simulink model "vehicle_model"  (R2021b)
settings: Solver=ode23tb  StartTime=0  StopTime=181.45  FixedStep=1e-5  RelTol=2e-1
InitFcn:
  | param_v1_script;
  | Ts=0.01;
  | scenario_generator;
  | Regen_on=0;
  | v_nom=10;
  | load('eq_udds.mat')
  | %load('eq_nedc.mat')
values from neighbouring files (symbols this model uses):
  b = 1.504    [dynamics_wheel.m]    (also in param_v1_script.m = Simulink.Parameter)
  BattChargeMax = 4.8    [param_v1_script.m]
  Battery = struct    [param_v1_script.m]
  BattSocInit = 0.75    [param_v1_script.m]
  BattTempInit = 25    [param_v1_script.m]
  BrkPrsMax = 5.0E+6    (= 5000000)    [param_v1_script.m]
  car = vehicle(scenario,'ClassID',1,'Position',[x_ego y_ego 0], 'Yaw' ,0,     'Length',3,'Width',2,'Height',1.6)    [scenario_generator.m]
  curvature = (DX.*D2Y - DY.*D2X) ./(DX.^2+DY.^2).^(3/2)    [ref_generator.m]
  direction = ones(length(gradbp),1)    [ref_generator.m]
  disk_abore = 0.05    [param_v1_script.m]
  Eb_init = 54.28*1000*3600    (= 195408000)    [param_v1_script.m]
  efficiency_table = [86.7 86.7 86.7 86.7 86.7 86.7 86.7 86.7 86.7 86.7 86.7 86.7 86.7 86.7     86.7 ... (first row only)    [param_v1_script.m]
  eta_i = 1    [param_v1_script.m]
  gradbp = distbp    [ref_generator.m]
  Jmotor = Simulink.Parameter    [param_v1_script.m]
  k = Simulink.Parameter    [param_v1_script.m]
  L = 30000    [scenario_generator.m]
  losses_table = [0 0 0 0 0 0 0 0 0 0 0 0 0 0 0 ... (first row only)    [param_v1_script.m]
  m = 3152    [param_v1_script.m]
  MaxChrgCurrLim = Simulink.Parameter    [param_v1_script.m]
  MaxDchrgCurrLim = Simulink.Parameter    [param_v1_script.m]
  MinCellVoltDchrgCurrentLim_BP = [2.5; 2.75; 3]    [param_v1_script.m]
  MinCellVoltDchrgCurrentLim_Table = [0 0.5 1]    [param_v1_script.m]
  MotSpd = [0 1600 3200 4477.56 4800 6400 8000 9600 11200 12800 14400 16000            ]    [param_v1_script.m]
  MotTrq = [450 450 450 450 419.771162404874 314.828371803655 251.862697442924            209.885581202437 179.901926744946 157.414185901828 139.923720801625            125.931348721462]    [param_v1_script.m]
  mu_kinetic = 0.2    [param_v1_script.m]
  Nd = 12    [param_v1_script.m]
  Ndiff = Simulink.Parameter    [param_v1_script.m]
  Np_Module = 31    [param_v1_script.m]
  Ns_Module = 24    [param_v1_script.m]
  num_pads = 2    [param_v1_script.m]
  NumModules = 4    [param_v1_script.m]
  psi_o = thetaRefs(1)*(pi/180)    [ref_generator.m]
  RegenBrkCutOff = [0 1]    [param_v1_script.m]
  RegenBrkSpd_bpt = [5 9]    [param_v1_script.m]
  Rm = 0.177    [param_v1_script.m]
  rw = 0.419    [param_v1_script.m]
  scenario = drivingScenario('SampleTime',0.1','StopTime',60)    [scenario_generator.m]
  SOCInit = 0.75    [param_v1_script.m]
  SOE_init = SOCInit    (= 0.75)    [param_v1_script.m]
  T_eff_bp = [0 32.142857142857146 64.285714285714292 96.428571428571431              128.57142857142858 160.71428571428572 192.85714285714286 225              257.14285714285717 289.28571428571428 321.42857142857144 353.57142857142856              385.71428571428572 417.85714285714283 450]    [param_v1_script.m]
  thetaRefs = smooth(gradbp,thetaRef)    [ref_generator.m]
  threshld = 50    [scenario_generator.m]
  VEH = struct    [dynamics_wheel.m]
  w_eff_bp = [0 1600 3200 4477.56 4800 6400 8000 9600 11200 12800 14400 16000              ]    [param_v1_script.m]
  xRef2s = smooth(gradbp,xRef2)    [ref_generator.m]
  yRef2s = smooth(gradbp,yRef2)    [ref_generator.m]
undefined symbols (not defined in the file or in its folder): DiscIntNeverNeededParam, InertFrm
libraries: simulink x11, autolibsharedcoupling x10, autolibshared x5, autolibutils x4, autolibshareddiff x3, sharedtransform x3, vehdynlibdriver x3, simulink_extras x3, sharedTrackingLibrary x2, vehdynlibtirecommon x2, vehdynlibtire x2, vehdynlibdrivercommon x2
(part 6 of 6)

== system vehicle_model/Passenger Car/Subsystem1/Subsystem1/Longitudinal Wheels 4DOF/Axle Forces/Bicycle/Wheel to Body Transform ==
  Forces : Inport  PortDimensions=[3,1]  Partition=on  PartitionDimension=2  PartitionWidth=1  PartitionOffset=0
  WheelAngles : Inport  Port=2  Partition=on  PartitionDimension=2  PartitionWidth=1  PartitionOffset=0
  Demux1 : Demux  Outputs=3
  Divide1 : Product  Inputs=**  Multiplication=Matrix(*)
  For Each : ForEach  DisableCoverage=on
  Rotation Angles to Direction Cosine Matrix : sharedtransform/Rotation Angles to Direction Cosine Matrix  rotationOrder=ZYX  aMode=2
      settings: SourceProductBaseCode=AE,PW,DR,MT,UV,VE
  Selector : Selector  InputPortWidth=3  IndexOptions=Index vector (dialog)  Indices=[3 2 1]  OutputSizes=1
  Fx : Outport  ConcatenationDimension=1  VectorParamsAs1DForOutWhenUnconnected=off
  Fy : Outport  Port=2  ConcatenationDimension=1  VectorParamsAs1DForOutWhenUnconnected=off
  Fz : Outport  Port=3  ConcatenationDimension=1  VectorParamsAs1DForOutWhenUnconnected=off
  wires:
  Selector/1 -> Rotation Angles to Direction Cosine Matrix/1
  WheelAngles/1 -> Selector/1
  Forces/1 -> Divide1/2
  Rotation Angles to Direction Cosine Matrix/1 -> Divide1/1
  Demux1/3 -> Fz/1
  Demux1/2 -> Fy/1
  Demux1/1 -> Fx/1
  Divide1/1 -> Demux1/1

== system vehicle_model/Passenger Car/Subsystem1/Subsystem1/Longitudinal Wheels 4DOF/Axle Forces/Dual/Wheel Angles ==
  Front : Inport
  Camber : Inport  Port=2
  Add1 : Sum
  Add2 : Sum
  Constant1 : Constant  Value=pi
  Constant2 : Constant  Value=[pi;0;pi;0].*0+[0;pi;0;pi].*.0
  Constant3 : Constant  Value=ones(1,4).*0
  Reshape : Reshape  OutputDimensionality=Row vector (2-D)
  Reshape1 : Reshape  OutputDimensionality=Row vector (2-D)
  Reshape2 : Reshape  OutputDimensionality=Row vector (2-D)
  Vector Concatenate3 : Concatenate  NumInputs=3  Mode=Multidimensional array
  Vehicle : Outport  VectorParamsAs1DForOutWhenUnconnected=off
  wires:
  Constant1/1 -> Add2/2
  Reshape/1 -> Vector Concatenate3/3
  Reshape2/1 -> Vector Concatenate3/2
  Front/1 -> Add1/1
  Add2/1 -> Reshape1/1
  Add1/1 -> Reshape/1
  Constant3/1 -> Reshape2/1
  Reshape1/1 -> Vector Concatenate3/1
  Constant2/1 -> Add1/2
  Camber/1 -> Add2/1
  Vector Concatenate3/1 -> Vehicle/1

== system vehicle_model/Passenger Car/Subsystem1/Subsystem1/Longitudinal Wheels 4DOF/Axle Forces/Dual/Wheel to Body Transform ==
  Forces : Inport  PortDimensions=[3,1]  Partition=on  PartitionDimension=2  PartitionWidth=1  PartitionOffset=0
  WheelAngles : Inport  Port=2  Partition=on  PartitionDimension=2  PartitionWidth=1  PartitionOffset=0
  Demux1 : Demux  Outputs=3
  Divide1 : Product  Inputs=**  Multiplication=Matrix(*)
  For Each : ForEach  DisableCoverage=on
  Rotation Angles to Direction Cosine Matrix : sharedtransform/Rotation Angles to Direction Cosine Matrix  rotationOrder=ZYX  aMode=2
      settings: SourceProductBaseCode=AE,PW,DR,MT,UV,VE
  Selector : Selector  InputPortWidth=3  IndexOptions=Index vector (dialog)  Indices=[3 2 1]  OutputSizes=1
  Fx : Outport  ConcatenationDimension=1  VectorParamsAs1DForOutWhenUnconnected=off
  Fy : Outport  Port=2  ConcatenationDimension=1  VectorParamsAs1DForOutWhenUnconnected=off
  Fz : Outport  Port=3  ConcatenationDimension=1  VectorParamsAs1DForOutWhenUnconnected=off
  wires:
  Divide1/1 -> Demux1/1
  Demux1/1 -> Fx/1
  Demux1/2 -> Fy/1
  Demux1/3 -> Fz/1
  Rotation Angles to Direction Cosine Matrix/1 -> Divide1/1
  Forces/1 -> Divide1/2
  WheelAngles/1 -> Selector/1
  Selector/1 -> Rotation Angles to Direction Cosine Matrix/1

== system vehicle_model/Passenger Car/Subsystem1/Subsystem1/Longitudinal Wheels 4DOF/Tires/MF/scale factors with friction ==
  lamda_mu_x : Inport
  lamda_mu_y : Inport  Port=2
  0 : Constant  Value=[zeros(1,numWheels)]  VectorParams1D=off
  Reshape : Reshape  OutputDimensionality=Row vector (2-D)  OutputDimensions=[1,numWheels]
  Reshape1 : Reshape  OutputDimensionality=Row vector (2-D)  OutputDimensions=[1,numWheels]
  Signal Specification3 : SignalSpecification  Unit=1
  Vector Concatenate : Concatenate  NumInputs=5  Mode=Multidimensional array
  ones : Constant  Value=[ones(23,numWheels)]  VectorParams1D=off
  ones2 : Constant  Value=ones(1,numWheels)  VectorParams1D=off
  lambdas : Outport  Unit=1  VectorParamsAs1DForOutWhenUnconnected=off
  wires:
  lamda_mu_y/1 -> Reshape1/1
  lamda_mu_x/1 -> Reshape/1
  ones2/1 -> Vector Concatenate/1  "lambda_Fz0"
  Vector Concatenate/1 -> Signal Specification3/1
  ones/1 -> Vector Concatenate/5
  0/1 -> Vector Concatenate/4  "lamda_mu_V"
  Reshape1/1 -> Vector Concatenate/3
  Reshape/1 -> Vector Concatenate/2
  Signal Specification3/1 -> lambdas/1

== system vehicle_model/Passenger Car/Subsystem1/Subsystem1/Longitudinal Wheels 4DOF/Velocity and Vertical Load/Bicycle/Bicycle Fz ==
  Bus Element In1 : Inport  PortName=VehFdbk
  Add : Sum
  Bus Selector : BusSelector  OutputSignals=BdyFrm.Forces.Tires.FrntTire.Fz,BdyFrm.Forces.Tires.RearTire.Fz
  Cont LPF : autolibutils/Cont LPF  wc=100*2*pi*ones(4,1)  aMode=2
      settings: SourceProductBaseCode=PW,DR,MT,UV,VE
  Saturation : Saturate  UpperLimit=10e3*ones(4,1)  LowerLimit=100*ones(4,1)  ZeroCross=off
  Unsprung Mass : Constant  Value=[0 0 80 80].*9.81
  Vector Concatenate : Concatenate  NumInputs=4
  Out1 : Outport  PortDimensions=4  VectorParamsAs1DForOutWhenUnconnected=off
  wires:
  Vector Concatenate/1 -> Saturation/1
  Saturation/1 -> Cont LPF/1
  Cont LPF/1 -> Add/1
  Bus Element In1/1 -> Bus Selector/1
  Bus Selector/1 -> Vector Concatenate/2, Vector Concatenate/1  "<Fz>"
  Bus Selector/2 -> Vector Concatenate/3, Vector Concatenate/4  "<Fz>"
  Unsprung Mass/1 -> Add/2
  Add/1 -> Out1/1

== system vehicle_model/Passenger Car/Subsystem1/Subsystem1/Longitudinal Wheels 4DOF/Velocity and Vertical Load/Bicycle/Bicycle V ==
  In1 : Inport
  Bus Selector : BusSelector  OutputSignals=BdyFrm.FrntAxl.Vel.xdot,BdyFrm.FrntAxl.Vel.ydot,BdyFrm.FrntAxl.Vel.zdot
  Bus Selector3 : BusSelector  OutputSignals=BdyFrm.RearAxl.Vel.xdot,BdyFrm.RearAxl.Vel.ydot,BdyFrm.RearAxl.Vel.zdot
  Mux : Mux  Inputs=3
  Mux1 : Mux  Inputs=3
  Vector Concatenate1 : Concatenate  NumInputs=4  Mode=Multidimensional array  ConcatenateDimension=2
  Out1 : Outport  PortDimensions=[3,4]  VectorParamsAs1DForOutWhenUnconnected=off
  wires:
  Bus Selector3/1 -> Mux1/1  "<xdot>"
  Mux/1 -> Vector Concatenate1/2, Vector Concatenate1/1
  In1/1 -> Bus Selector3/1, Bus Selector/1
  Bus Selector/1 -> Mux/1  "<xdot>"
  Mux1/1 -> Vector Concatenate1/4, Vector Concatenate1/3
  Vector Concatenate1/1 -> Out1/1
  Bus Selector/2 -> Mux/2  "<ydot>"
  Bus Selector/3 -> Mux/3  "<zdot>"
  Bus Selector3/2 -> Mux1/2  "<ydot>"
  Bus Selector3/3 -> Mux1/3  "<zdot>"

== system vehicle_model/Passenger Car/Subsystem1/Subsystem1/Longitudinal Wheels 4DOF/Velocity and Vertical Load/Dual/Dual Fz ==
  In1 : Inport
  Add : Sum
  Bus Selector6 : BusSelector  OutputSignals=BdyFrm.Forces.Tires.FrntTires.Lft.Fz,BdyFrm.Forces.Tires.FrntTires.Rght.Fz,BdyFrm.Forces.Tires.RearTires.Lft.Fz,BdyFrm.Forces.Tires.RearTires.Rght.Fz
  Cont LPF : autolibutils/Cont LPF  wc=100*2*pi  aMode=2
      settings: SourceProductBaseCode=PW,DR,MT,UV,VE
  Saturation : Saturate  UpperLimit=10e3  LowerLimit=100  ZeroCross=off
  Unsprung Mass : Constant  Value=[0 0 80 80].*9.81
  Vector Concatenate : Concatenate  NumInputs=4
  Out1 : Outport  VectorParamsAs1DForOutWhenUnconnected=off
  wires:
  In1/1 -> Bus Selector6/1
  Saturation/1 -> Cont LPF/1
  Cont LPF/1 -> Add/1
  Vector Concatenate/1 -> Saturation/1
  Bus Selector6/2 -> Vector Concatenate/2  "<Fz>"
  Bus Selector6/1 -> Vector Concatenate/1  "<Fz>"
  Bus Selector6/3 -> Vector Concatenate/3  "<Fz>"
  Bus Selector6/4 -> Vector Concatenate/4  "<Fz>"
  Add/1 -> Out1/1
  Unsprung Mass/1 -> Add/2

== system vehicle_model/Passenger Car/Subsystem1/Subsystem1/Longitudinal Wheels 4DOF/Velocity and Vertical Load/Dual/Dual V ==
  In1 : Inport
  Bus Selector1 : BusSelector  OutputSignals=BdyFrm.FrntAxl.Lft.Vel.xdot,BdyFrm.FrntAxl.Lft.Vel.ydot,BdyFrm.FrntAxl.Lft.Vel.zdot  OutputAsBus=on
  Bus Selector2 : BusSelector  OutputSignals=BdyFrm.FrntAxl.Rght.Vel.xdot,BdyFrm.FrntAxl.Rght.Vel.ydot,BdyFrm.FrntAxl.Rght.Vel.zdot  OutputAsBus=on
  Bus Selector4 : BusSelector  OutputSignals=BdyFrm.RearAxl.Lft.Vel.xdot,BdyFrm.RearAxl.Lft.Vel.ydot,BdyFrm.RearAxl.Lft.Vel.zdot  OutputAsBus=on
  Bus Selector5 : BusSelector  OutputSignals=BdyFrm.RearAxl.Rght.Vel.xdot,BdyFrm.RearAxl.Rght.Vel.ydot,BdyFrm.RearAxl.Rght.Vel.zdot  OutputAsBus=on
  Bus to Vector{5..8} (4 alike) : BusToVector
  Vector Concatenate2 : Concatenate  NumInputs=4  Mode=Multidimensional array  ConcatenateDimension=2
  Out1 : Outport  VectorParamsAs1DForOutWhenUnconnected=off
  wires:
  Bus to Vector6/1 -> Vector Concatenate2/2
  Bus Selector2/1 -> Bus to Vector6/1
  Bus to Vector8/1 -> Vector Concatenate2/4
  Bus Selector4/1 -> Bus to Vector7/1
  Bus to Vector5/1 -> Vector Concatenate2/1
  Bus Selector1/1 -> Bus to Vector5/1
  In1/1 -> Bus Selector1/1, Bus Selector2/1, Bus Selector4/1, Bus Selector5/1
  Bus Selector5/1 -> Bus to Vector8/1
  Bus to Vector7/1 -> Vector Concatenate2/3
  Vector Concatenate2/1 -> Out1/1

== matlab function vehicle_model/Subsystem2/MATLAB Function ==
  data: Tm input; Pb output; wm input
function Pb = fcn(Tm, wm)
c1=2.238e-11; c2=-2.627e-14; c3= 8.637e-14; c4=2.062e-19; c5=1; 
Pb=(c1+c2*wm+c3*Tm+c4*wm^2+c5*wm*Tm);

== matlab function vehicle_model/Passenger Car/Subsystem1/Subsystem1/Vehicle Signal Routing/For 3D Visualization ==
  data: angles output size=3; angleIn input size=3; GeomXYZ output size=3; GemoXYZIn input size=3; Ground input size=4; trackW parameter; wheelB parameter
function [angles,GeomXYZ]= three26(angleIn, GemoXYZIn, Ground,trackW, wheelB)%#codegen
coder.allowpcode('plain')
% Copyright 2018 The MathWorks, Inc.
[angles,GeomXYZ]= vdynthree2six(angleIn, GemoXYZIn, Ground,trackW, wheelB);
